simulink model "IEEE13bus_1subsystem"  (R2022b)
settings: Solver=ode4  StartTime=0.0  StopTime=inf  FixedStep=Ts  MaxStep=1e-4  RelTol=1e-4
InitFcn:
  | a=1; % Loading Factor
  | Ts=50e-6;
  | % phase to sequence conversion of RXB matrices
  | c=1*exp(sqrt(-1)*(120*pi/180));
  | T=[1 1 1;1 c*c c;1 c c*c];
  | Tinv=1/3*[1 1 1;1 c c*c;1 c*c c];
  | 
  | % Simulation data for the IEEE 13 Node Test Feeder model
  | mi2km = 1.60934;%  miles to km conversion
  | ft2km = 0.0003048; % feet to km conversion
  | ms2F = 1*1e-6/(2*pi*60);% microsiemens to Farads conversion
  | 
  | 
  | %% Configuration 601
  | % Series Resitance and Reactance - ohm/mile
  | R_601 = [0.3465 0.1560 0.1580;0.1560 0.3375 0.1535;0.1580 0.1535 0.3414];
  | X_601 = [1.1079 0.5017 0.4236;0.5017 1.0478 0.3849;0.4236 0.3849 1.0348];
  | % charging susceptance - microsiemens/mile
  | B_601 = [6.2998 -1.9958 -1.2595;-1.9958 5.9597 -0.7417;-1.2595 -0.7417 5.6386];
  | 
  | R_601 = R_601/mi2km;
  | Rseq=Tinv*R_601*T;
  | R1_601=Rseq(2,2);R0_601=Rseq(1,1);
  | 
  | L_601 = (X_601/(2*pi*60))/mi2km;
  | Lseq=Tinv*L_601*T;
  | L1_601=Lseq(2,2);L0_601=Lseq(1,1);
  | 
  | C_601 =(B_601*ms2F)/mi2km;
  | Cseq=Tinv*C_601*T;
  | C1_601=Cseq(2,2);C0_601=Cseq(1,1);
  | 
  | %% Configuration 602 - series reactance - ohm/mile
  | R_602 = [0.7526 0.1580 0.1560;0.1580 0.7475 0.1535;0.1560 0.1535 0.7436];
  | X_602 = [1.1814 0.4236 0.5017;0.4236 1.1983 0.3849;0.5017 0.3849 1.2112];
  | % charging susceptance - microsiemens/mile
  | B_602 = [5.6990 -1.0817 -1.6905;-1.0817 5.1795 -0.6588;-1.6905 -0.6588 5.4246];
  | 
  | R_602 = R_602/mi2km;
  | Rseq=Tinv*R_602*T;
  | R1_602=Rseq(2,2);R0_602=Rseq(1,1);
  | 
  | L_602 = (X_602/(2*pi*60))/mi2km;
  | Lseq=Tinv*L_602*T;
  | L1_602=Lseq(2,2);L0_602=Lseq(1,1);
  | 
  | C_602 =(B_602*ms2F)/mi2km;
  | Cseq=Tinv*C_602*T;
  | C1_602=Cseq(2,2);C0_602=Cseq(1,1);
  | %% Configuration 603 - series reactance - ohm/mile
  | R_603 = [0 0 0;0 1.3294 0.2066;0 0.2066 1.3238];
  | X_603 = [0 0 0;0 1.3471 0.4591;0 0.4591 1.3569];
  | % charging susceptance - microsiemens/mile
  | B_603 = [0 0 0;0 4.7097 -0.8999;0 -0.8999 4.6658];
  | 
  | % convert for SPS
  | R_603 = R_603/mi2km;
  | Rseq=Tinv*R_603*T;
  | R1_603=Rseq(2,2);R0_603=Rseq(1,1);
  | 
  | L_603 = (X_603/(2*pi*60))/mi2km;
  | Lseq=Tinv*L_603*T;
  | L1_603=Lseq(2,2);L0_603=Lseq(1,1);
  | 
  | C_603 =(B_603*ms2F)/mi2km;
  | Cseq=Tinv*C_603*T;
  | C1_603=Cseq(2,2);C0_603=Cseq(1,1);
  | %% Configuration 604 - series reactance - ohm/mile
  | R_604 = [1.3238 0 0.2066;0 0 0;0.2066 0 1.3294];
  | X_604 = [1.3569 0 0.4591;0 0 0;0.4591 0 1.3471];
  | % charging susceptance - microsiemens/mile
  | B_604 = [4.6658 0 -0.8999;0 0 0;-0.8999 0 4.7097];
  | R_604 = R_604/mi2km;
  | Rseq=Tinv*R_604*T;
  | R1_604=Rseq(2,2);R0_604=Rseq(1,1);
  | 
  | L_604 = (X_604/(2*pi*60))/mi2km;
  | Lseq=Tinv*L_604*T;
  | L1_604=Lseq(2,2);L0_604=Lseq(1,1);
  | 
  | C_604 =(B_604*ms2F)/mi2km;
  | Cseq=Tinv*C_604*T;
  | C1_604=Cseq(2,2);C0_604=Cseq(1,1);
  | %% Configuration 605 - series reactance - ohm/mile
  | R_605 = [0 0 0;0 0 0;0 0 1.3292];
  | X_605 = [0 0 0;0 0 0;0 0 1.3475];
  | % charging susceptance - microsiemens/mile
  | B_605 = [0 0 0;0 0 0;0 0 4.5193];
  | R_605 = R_605/mi2km;
  | Rseq=Tinv*R_605*T;
  | R1_605=Rseq(2,2);R0_605=Rseq(1,1);
  | 
  | L_605 = (X_605/(2*pi*60))/mi2km;
  | Lseq=Tinv*L_605*T;
  | L1_605=Lseq(2,2);L0_605=Lseq(1,1);
  | 
  | C_605 =(B_605*ms2F)/mi2km;
  | Cseq=Tinv*C_605*T;
  | C1_605=Cseq(2,2);C0_605=Cseq(1,1);
  | %% Configuration 606 - series reactance - ohm/mile
  | R_606 = [0.7982 0.3192 0.2849;0.3192 0.7891 0.3192;0.2849 0.3192 0.7982];
  | X_606 = [0.4463 0.0328 0.0143;0.0328 0.4041 0.0328;0.0143 0.0328 0.4463];
  | % charging susceptance - microsiemens/mile
  | B_606 = [96.8897 -1e-6 -1e-6;-1e-6 96.8897 -1e-6;-1e-6 -1e-6 96.8897];
  | R_606 = R_606/mi2km;
  | Rseq=Tinv*R_606*T;
  | R1_606=Rseq(2,2);R0_606=Rseq(1,1);
  | 
  | L_606 = (X_606/(2*pi*60))/mi2km;
  | Lseq=Tinv*L_606*T;
  | L1_606=Lseq(2,2);L0_606=Lseq(1,1);
  | 
  | C_606 =(B_606*ms2F)/mi2km;
  | Cseq=Tinv*C_606*T;
  | C1_606=Cseq(2,2);C0_606=Cseq(1,1);
  | %% Configuration 607 - series reactance - ohm/mile
  | R_607 = [1.3425 0 0;0 0 0;0 0 0];
  | X_607 = [0.5124 0 0;0 0 0;0 0 0];
  | % charging susceptance - microsiemens/mile
  | B_607 = [88.9912 0 0;0 0 0;0 0 0];
  | R_607 = R_607/mi2km;
  | Rseq=Tinv*R_607*T;
  | R1_607=Rseq(2,2);R0_607=Rseq(1,1);
  | 
  | L_607 = (X_607/(2*pi*60))/mi2km;
  | Lseq=Tinv*L_607*T;
  | L1_607=Lseq(2,2);L0_607=Lseq(1,1);
  | 
  | C_607 =(B_607*ms2F)/mi2km;
  | Cseq=Tinv*C_607*T;
  | C1_607=Cseq(2,2);C0_607=Cseq(1,1);
undefined symbols (not defined in the file): find_system, I, Left, MOV_segment9, powergui, Right, type, V, X
libraries: spsSeriesRLCBranchLib x57, spsGroundLib x42, spsVoltageMeasurementLib x18, spsThreePhaseVIMeasurementLib x16, spsDCVoltageSourceLib x12, spsThreePhaseSeriesRLCLoadLib x7, ssn_lib x6, spsACCurrentSourceLib x6, spsOnDelayLib x6, spsThreePhasePISectionLineLib x5, spsSeriesRLCLoadLib x5, spsRMSLib x4
(part 1 of 4)
settings Model: ARTEMISmethode_block_infos=$$__separator__$$IEEE13bus_1subsystem/ARTEMIS Guide$$__separator__$$  Creator=Arun  LastModifiedBy=AS7434
settings SolverCC: ShapePreserveControl=EnableAll  AlgebraicLoopSolver=TrustRegion  SolverResetMethod=Robust
settings DataIOCC: ReturnWorkspaceOutputs=off
settings DebuggingCC: SFMachineParentedDataDiag=warning  ArithmeticOperatorsInVariantConditions=warning
settings ModelReferenceCC: EnableRefExpFcnMdlSchedulingChecks=on
settings SFSimCC: SimUseLocalCustomCode=off  CustomCodeUndefinedFunction=UseInterfaceOnly
settings RTWCC: RTWUseLocalCustomCode=off
settings CodeAppCC: StateflowObjectComments=on
settings SimscapeCC: SimscapeNormalizeSystem=off

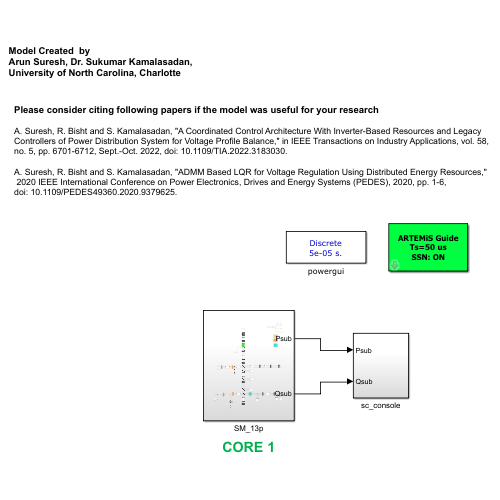
[thumbnail: Simulink's stored preview of the top-level diagram]
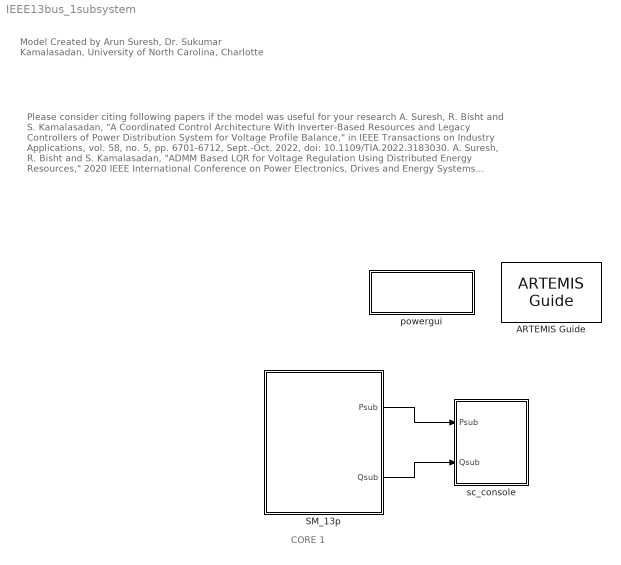
== system IEEE13bus_1subsystem ==
  note: CORE 1
  note: Please consider citing following papers if the model was useful for your research
      |
      | A. Suresh, R. Bisht and S. Kamalasadan, "A Coordinated Control Architecture With Inverter-Based Resources and Legacy
      | Controllers of Power Distribution System for Voltage Profile Balance," in IEEE Transactions on Industry Applications, vol. 58,
      | no. 5, pp. 6701-6712, Sept.-Oct. 2022, doi: 10.1109/TIA.2022.3183030.
      |
      | A. Suresh, R. Bisht and S. Kamalasadan, "ADMM Based LQR for Voltage Regulation Using Distributed Energy Resources,"
      | 2020 IEEE International Conference on Power Electronics, Drives and Energy Systems (PEDES), 2020, pp. 1-6,
      | doi: 10.1109/PEDES49360.2020.9379625.
  note: Model Created by
      | Arun Suresh, Dr. Sukumar Kamalasadan,
      | University of North Carolina, Charlotte
  ARTEMIS Guide : artemis/ARTEMIS/ARTEMIS Guide  Tag=FTSSmethode_opal_4hx0r99  Description=5.0_z1  lock=on  Ts=Ts  ssn=on  opt=art5  dyna=off  nb_perm=4  RT_fullcomp=off  ssn_itvc=off  ssn_ivic=off  ssn_ext=off  ssn_solver=Art5  iter_type=iSWITCH and iMOV only (default)  ssn_ImpulseLoopBlockedStateUpdate=5  ssn_mov_iter_number=5  ssn_switch_iter_number=5  ssn_lu_or_ldlt=LU (more robust)  ssn_nib_type_verify=on  ssn_use_lu=on  ssn_use_ldlt=off  ssn_impulse=on  ssn_quasimpulse=off  ssn_impulse_loop=5  paraExtinctionThy=off  Thy_Impulse=on  dtc=Off  dtc_opt=normal  ao=on  simtype=off  ct_mac=off  lin_mov=off  lsp=[0.001 2]  spike_skip=Disabled  dtc_extra=1  dtc_sws=normal  dtc_pied=0.5  SPSRulesBlock=SPSRules  tre=on  ctmm=off  LF=off  dpl_type=ARTEMiS DPL  rlc_type=off  custom_type=off  para=on  ssn_full_iteration=off  ssn_init_cond=block only
  SM_13p : Subsystem
  powergui : Subsystem  Priority=1  DialogController=POWERSYS.PowerSysDialog  InitFcn=powergui( 'InitFcn_Callback' , gcb , 0 , [ ] );  mask(PSB option menu block){SimulationMode=Discrete, SampleTime=Ts, frequency=60, Iterations=50, frequencyindice=0, Pbase=100e6, ErrMax=1e-4, UnitsV=kV, UnitsW=MW, buscounter=0, FunctionMessages=off, echomessages=on, EnableUseOfTLC=off, CurrentSourceSwitches=off, DisableSnubberDevices=off, DisableRonSwitches=off, DisableVfSwitches=off, DisplayEquations=off, AutomaticDiscreteSolvers=off, SolverType=Tustin, Interpol=off, ExternalGateDelay=off, methode=off, Ts=0, x0status=blocks, SPID=off, SwTol=0, HookPort=off, NonlinearTolerance=1e-4, nMaxIteration=100, ContinueOnMaxIteration=off, RestoreLinks=warning, ResistiveCurrentMeasurement=off, Frange=[0:2:500], Ylog=off, Xlog=on, ShowGrid=off, save=off, variable=ZData, structure=0, ZoomFFT=off, StartTime=0.0, cycles=1, DisplayStyle=1, fundamental=60, FreqAxis=off, MaxFrequency=1000, frequencyindicesteady=1, RmsSteady=1, display=off}
      mask prompts: SimulationMode "Simulation type:"; SampleTime "Sample time (s):"; frequency "Frequency (Hz):"; Iterations "Max iterations"; frequencyindice "Frequency (Hz)"; Pbase "Base power (VA)"; ErrMax "PQ tolerance (pu)"; UnitsV "Voltage units"; UnitsW "Power units"; buscounter "Load flow bus counter"; FunctionMessages "Disable Specialized Power Systems warnings"; echomessages "Display Specialized Power Systems compilation messages"; EnableUseOfTLC "Use TLC file when in Accelerator Simulation Mode and for code generation"; CurrentSourceSwitches "Disable ideal switching"; DisableSnubberDevices "Disable snubbers in switching devices"; DisableRonSwitches "Disable Ron resistances in switching devices"; DisableVfSwitches "Disable forward voltages in switching devices"; DisplayEquations "Display circuit differential equations"; AutomaticDiscreteSolvers "Automatically handle Discrete solver and Advanced tab solver settings of blocks"; SolverType "Discrete solver"; Interpol "Interpolate switching events"; ExternalGateDelay "Use time-stamped gate signals"; methode "Store switching topologies"; Ts "Buffer size (MBytes):"; x0status "Start simulation with initial electrical states from:"; SPID "Use ideal switching devices"; SwTol "Switch tolerance"; HookPort "Allow multiple powergui blocks"; NonlinearTolerance "Solver tolerance"; nMaxIteration "Maximum number of iterations"; ContinueOnMaxIteration "Continue Simulation if maximum number of iterations is reached"; RestoreLinks "Restore disabled links of Simscape Power Systems ST blocks:"; ResistiveCurrentMeasurement "Use non ideal current measurement blocks (1e-4Ohm internal resistance)"; Frange "Frequency Range"; Ylog "Log impedance"; Xlog "log Frequency"; ShowGrid "grid"; save "Save Data To Workspace"; variable "Variable Name"; structure "Structure Name (PSBFFTSCOPE)"; ZoomFFT "ZoomFFT (PSBFFTSCOPE)"; StartTime "Start Time (PSBFFTSCOPE)"; cycles "Cycles (PSBFFTSCOPE)"; DisplayStyle "Display style (PSBFFTSCOPE)"; fundamental "Fundamental (PSBFFTSCOPE)"; FreqAxis "Frequency Axis (PSBFFTSCOPE)"; MaxFrequency "Max Frequency (PSBFFTSCOPE)"; frequencyindicesteady "Frequency indice (STEADYSTATE)"; RmsSteady "RMS display (STEADYSTATE)"; display "Display Results"
      mask help: Set simulation type, simulation parameters, and preferences.
      mask init:
      | dispMessage = powergui('MaskInitialization',gcb,SimulationMode,SampleTime);
      settings: LibrarySourceBlock=sps_lib/powergui  PreSaveFcn=powergui( 'PreSaveFcn_Callback' , gcb , [ ] , [ ] );  OpenFcn=sps_rtmsupport('OpenFcn',gcbh)
      mask Help: helpview(psbhelp)
      mask TypeOptions SimulationMode: Continuous | Discrete | Phasor | Discrete phasor
      mask Callback SimulationMode: powergui('SimulationType',[],[],gcb);
      mask TypeOptions UnitsV: V | kV
      mask TypeOptions UnitsW: W | kW | MW
      mask Callback CurrentSourceSwitches: powergui('SimulationType',[],[],gcb);
      mask Callback AutomaticDiscreteSolvers: powergui('SimulationType',[],[],gcb);
      mask TypeOptions SolverType: Tustin/Backward Euler (TBE) | Tustin | Backward Euler
      mask Callback SolverType: powergui('SimulationType',[],[],gcb);
      mask Callback Interpol: powergui('SimulationType',[],[],gcb);
      mask Callback ExternalGateDelay: powergui('SimulationType',[],[],gcb);
      mask Callback methode: powergui('SimulationType',[],[],gcb);
      mask TypeOptions x0status: blocks | steady | zero
      mask TypeOptions RestoreLinks: yes | warning | no
      mask Callback display: sps_rtmsupport('parametereditingmodes',gcbh) % Will be executed last in parameter callbacks to ensure mask enable consistency
      mask DialogControl SolverTab Prompt: Solver
      mask DialogControl AutoSolverNote Prompt: The Simulation type parameter is governed by Simulink. To access the Powergui solver settings, unselect auto (Automatic solver selection) solver in the Simulink solver options.
      mask DialogControl Container15 Prompt: Tools
      mask DialogControl StateAnalyzer Prompt: Measurements and States Analyzer
      mask DialogControl StateAnalyzer Callback: powerStates(bdroot(gcb))
      mask DialogControl RLCLineParameters Prompt: Power Line Parameters
      mask DialogControl RLCLineParameters Callback:
      | close_system(gcb)
      | powerLineParameters
      mask DialogControl Control15 Prompt: Power Cable Parameters
      mask DialogControl Control15 Callback:
      | close_system(gcb)
      | powerCableParameters
      mask DialogControl DecouplingLines Prompt: Specify Decoupling Lines
      mask DialogControl DecouplingLines Tooltip: Click to replace selected Distributed Parameters Line blocks with Decoupling Line blocks
      mask DialogControl DecouplingLines Callback:
      | close_system(gcb);
      | DecouplingLineReplace(gcs)
      mask DialogControl LoadFlow Prompt: Load Flow Analyzer
      mask DialogControl LoadFlow Callback:
      | close_system(gcb)
      | powerLoadFlow
      mask DialogControl Container11 Prompt: Load Flow Parameters
      mask DialogControl MachineInitialization Prompt: Machine Initialization
      mask DialogControl MachineInitialization Callback:
      | close_system(gcb)
      | powericon('machineInitTool',bdroot(gcb),gcb)
      mask DialogControl ImpedanceMeasurement Prompt: Impedance Measurement
      mask DialogControl ImpedanceMeasurement Callback:
      | close_system(gcb);
      | powerImpedance(bdroot(gcs));
      mask DialogControl FFTAnalysis Prompt: FFT Analysis
      mask DialogControl FFTAnalysis Callback:
      | close_system(gcb)
      | power_fftscope(bdroot(gcb),gcb)
      mask DialogControl LinearSystemAnalyzer Prompt: Use Linear System Analyzer
      mask DialogControl LinearSystemAnalyzer Callback:
      | close_system(gcb)
      | power_ltiview(bdroot(gcb))
      mask DialogControl HysteresisDesign Prompt: Hysteresis Design
      mask DialogControl HysteresisDesign Callback:
      | close_system(gcb)
      | powerHysteresis('hysteresis.mat')
      mask DialogControl Control14 Prompt: Customize SPS blocks
      mask DialogControl Control14 Callback:
      | close_system(gcb);
      | power_customize;
      mask DialogControl GenerateReprot Prompt: Generate Report
      mask DialogControl GenerateReprot Callback:
      | close_system(gcb)
      | power_report(bdroot(gcb))
      mask DialogControl ParameterTabVar012 Prompt: Preferences
      mask DialogControl Solver Prompt: Solver
      mask DialogControl SolverDetails Prompt: Solver details for nonlinear elements
      mask Display: color('blue'),disp(dispMessage)
  sc_console : Subsystem
  wires:
  SM_13p/1(Psub) -> sc_console/1(Psub)
  SM_13p/2(Qsub) -> sc_console/2(Qsub)

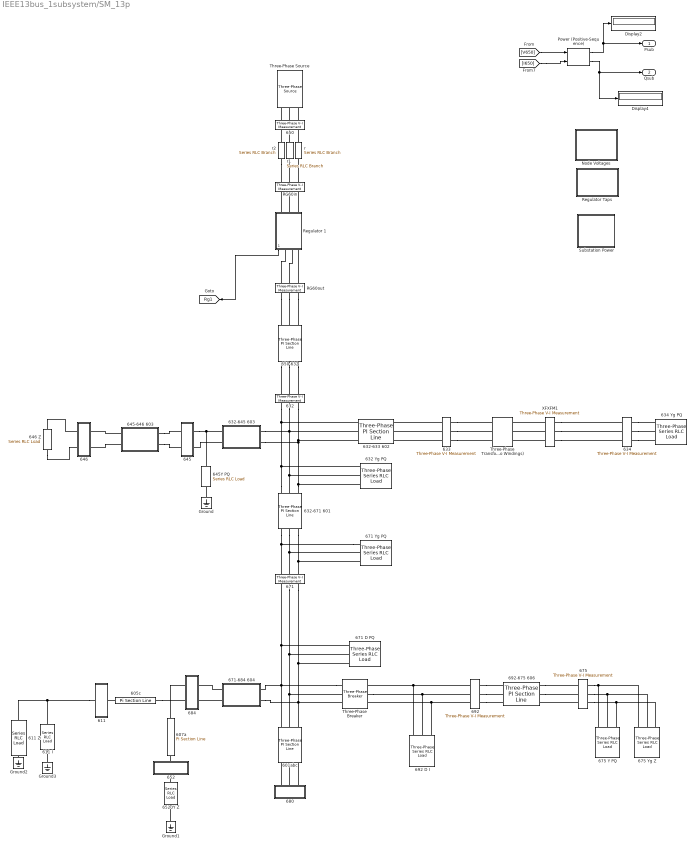
== system IEEE13bus_1subsystem/SM_13p ==
  601abc : spsThreePhasePISectionLineLib/Three-Phase PI Section Line  LConnTagsString=a|b|c  RConnTagsString=A|B|C  Length=1000*ft2km  Frequency=60  Resistances=[R1_601 R0_601]  Inductances=[L1_601 L0_601]  Capacitances=[C1_601 C0_601]
  605c : spsPiSectionLineLib/Pi Section Line  LConnTagsString=__new0  RConnTagsString=__new0  Phases=1  PiSections=1  Length=300*ft2km  Frequency=60  Resistance=R1_605  Inductance=L1_605  Capacitance=C1_605  SpecifyConductance=off  Conductance=0  Measurements=None  Measurements2=None
      settings: LibrarySourceBlock=sps_lib/Power Grid Elements/Pi Section Line
  607a : spsPiSectionLineLib/Pi Section Line  LConnTagsString=__new0  RConnTagsString=__new0  Phases=1  PiSections=1  Length=800*ft2km  Frequency=60  Resistance=R1_607  Inductance=L1_607  Capacitance=C1_607  SpecifyConductance=off  Conductance=0  Measurements=None  Measurements2=None
      settings: LibrarySourceBlock=sps_lib/Power Grid Elements/Pi Section Line
  611 : Subsystem
  611 I : spsSeriesRLCLoadLib/Series RLC Load  LConnTagsString=a  RConnTagsString=__new0  NominalVoltage=1*2401.78  NominalFrequency=60  ActivePower=170e3*a  InductivePower=80e3*a  CapacitivePower=0  Setx0=off  InitialVoltage=0  SetiL0=off  InitialCurrent=0  Measurements=None  LoadType=constant I
  611 Z : spsSeriesRLCLoadLib/Series RLC Load  LConnTagsString=a  RConnTagsString=__new0  NominalVoltage=2401.78  NominalFrequency=60  ActivePower=0  InductivePower=0  CapacitivePower=100e3*a  Setx0=off  InitialVoltage=0  SetiL0=off  InitialCurrent=0  Measurements=None  LoadType=constant Z
  632 : spsThreePhaseVIMeasurementLib/Three-Phase V-I Measurement  VoltageMeasurement=phase-to-ground  SetLabelV=on  LabelV=V632  Vpu=off  VpuLL=off  CurrentMeasurement=yes  SetLabelI=on  LabelI=I632  Ipu=off  Pbase=100e6  Vbase=24900  OutputType=Complex  PhasorSimulation=off  PSBequivalent=0
  632 Yg PQ : spsThreePhaseSeriesRLCLoadLib/Three-Phase Series RLC Load  LConnTagsString=A|B|C  Configuration=Y (grounded)  NominalVoltage=[ 1.021 1.042 1.0174]*2401.78  Vabc=[ 1 1 1]*2401.78  Vabcp=[1e3 1e3 1e3]  NominalFrequency=60  UnbalancedPower=on  ActivePower="[17 66  117]*1e3/2"  InductivePower="[10 38  68]*1e3/2"  CapacitivePower=100  Pabc="[17 66  117]*1e3/2*a"  QLabc="[10 38  68]*1e3/2*a"  QCabc=[0 0 0]  Pabcp=[10e3 9e3 11e3]  QLabcp=[100 90 110]  QCabcp=[100 90 110]  Measurements=None  LoadType=constant PQ
  632-633 602 : spsThreePhasePISectionLineLib/Three-Phase PI Section Line  LConnTagsString=a|b|c  RConnTagsString=A|B|C  Length=500*ft2km  Frequency=60  Resistances=[R1_602 R0_602]  Inductances=[L1_602 L0_602]  Capacitances=[C1_602 C0_602]
  632-645 603 : Subsystem  mask(Two-Phase PI Section Block){Rl=R_603, Ll=L_603, Cl=C_603, L=500*ft2km}
      mask prompts: Rl "Resistance per unit Length(Ohm/Km)[3x3 matrix]"; Ll "Inductance per unit Length(H/Km)[3x3 matrix]"; Cl "Capacitance per unit Length(F/Km)[3x3 matrix"; L "Length (Km)"
      mask help: This block models a two-phase transmission line with a single PI section.
      mask init:
      | W = sign(sum(abs(Rl)));
      | s = find(W==1);%Identify non zero rows and columns
      | 
      | Rt =Rl(s,s);
      | Rl= Rt;
      | Lt =Ll(s,s);
      | Ll= Lt;
      | Ct =Cl(s,s);
      | Cl= Ct;
      mask Display:
      | color('green')
      | plot(0,0,100,100,[20,20,80,80,90,80,80,20,20,10],[50,40,40,50,50,50,61,61,50,50],[56,39],[55,55],[44,44],[44,55],[53,50,50],[44,48,55])
      | color('black')
      | port_label('RConn', 1, 'b')
      | port_label('RConn', 2, 'c')
      | port_label('LConn', 1, 'B')
      | port_label('LConn', 2, 'C')
  632-671 601 : spsThreePhasePISectionLineLib/Three-Phase PI Section Line  LConnTagsString=a|b|c  RConnTagsString=A|B|C  Length=2000*ft2km  Frequency=60  Resistances=[R1_601 R0_601]  Inductances=[L1_601 L0_601]  Capacitances=[C1_601 C0_601]
  633 : spsThreePhaseVIMeasurementLib/Three-Phase V-I Measurement  VoltageMeasurement=phase-to-ground  SetLabelV=on  LabelV=V633  Vpu=off  VpuLL=off  CurrentMeasurement=no  SetLabelI=on  LabelI=I634  Ipu=off  Pbase=100e6  Vbase=24900  OutputType=Complex  PhasorSimulation=off  PSBequivalent=0
  634 : spsThreePhaseVIMeasurementLib/Three-Phase V-I Measurement  VoltageMeasurement=phase-to-ground  SetLabelV=on  LabelV=V634  Vpu=off  VpuLL=off  CurrentMeasurement=yes  SetLabelI=on  LabelI=I634  Ipu=off  Pbase=100e6  Vbase=24900  OutputType=Complex  PhasorSimulation=off  PSBequivalent=0
  634 Yg PQ : spsThreePhaseSeriesRLCLoadLib/Three-Phase Series RLC Load  LConnTagsString=A|B|C  Configuration=Y (grounded)  NominalVoltage=[ 1.021 1.042 1.0174]*2401.78  Vabc=[1 1 1]*277.128  Vabcp=[1e3 1e3 1e3]  NominalFrequency=60  UnbalancedPower=on  ActivePower="[17 66  117]*1e3/2"  InductivePower="[10 38  68]*1e3/2"  CapacitivePower=100  Pabc=[160 120 120]*1e3*a  QLabc=[110 90 90]*1e3*a  QCabc=[0 0 0]  Pabcp=[10e3 9e3 11e3]  QLabcp=[100 90 110]  QCabcp=[100 90 110]  Measurements=None  LoadType=constant PQ
  645 : Subsystem
  645-646 603 : Subsystem  mask(Two-Phase PI Section Block){Rl=R_603, Ll=L_603, Cl=C_603, L=300*ft2km}
      mask prompts: Rl "Resistance per unit Length(Ohm/Km)[3x3 matrix]"; Ll "Inductance per unit Length(H/Km)[3x3 matrix]"; Cl "Capacitance per unit Length(F/Km)[3x3 matrix"; L "Length (Km)"
      mask help: This block models a two-phase transmission line with a single PI section.
      mask init:
      | W = sign(sum(abs(Rl)));
      | s = find(W==1);%Identify non zero rows and columns
      | 
      | Rt =Rl(s,s);
      | Rl= Rt;
      | Lt =Ll(s,s);
      | Ll= Lt;
      | Ct =Cl(s,s);
      | Cl= Ct;
      mask Display:
      | color('green')
      | plot(0,0,100,100,[20,20,80,80,90,80,80,20,20,10],[50,40,40,50,50,50,61,61,50,50],[56,39],[55,55],[44,44],[44,55],[53,50,50],[44,48,55])
      | color('black')
      | port_label('RConn', 1, 'b')
      | port_label('RConn', 2, 'c')
      | port_label('LConn', 1, 'B')
      | port_label('LConn', 2, 'C')
  645Y PQ : spsSeriesRLCLoadLib/Series RLC Load  LConnTagsString=a  RConnTagsString=__new0  NominalVoltage=1*2401.78  NominalFrequency=60  ActivePower=170e3*a  InductivePower=125e3*a  CapacitivePower=0  Setx0=off  InitialVoltage=0  SetiL0=off  InitialCurrent=0  Measurements=None  LoadType=constant PQ
  646 : Subsystem
  646 Z : spsSeriesRLCLoadLib/Series RLC Load  LConnTagsString=a  RConnTagsString=__new0  NominalVoltage=4160  NominalFrequency=60  ActivePower=230e3*a  InductivePower=132e3*a  CapacitivePower=0  Setx0=off  InitialVoltage=0  SetiL0=off  InitialCurrent=0  Measurements=None  LoadType=constant Z
  650 : spsThreePhaseVIMeasurementLib/Three-Phase V-I Measurement  VoltageMeasurement=phase-to-ground  SetLabelV=on  LabelV=V650  Vpu=off  VpuLL=off  CurrentMeasurement=yes  SetLabelI=on  LabelI=I650  Ipu=off  Pbase=100e6  Vbase=24900  OutputType=Complex  PhasorSimulation=off  PSBequivalent=0
  650-632 : spsThreePhasePISectionLineLib/Three-Phase PI Section Line  LConnTagsString=a|b|c  RConnTagsString=A|B|C  Length=2000*ft2km  Frequency=60  Resistances=[R1_601 R0_601]  Inductances=[L1_601 L0_601]  Capacitances=[C1_601 C0_601]
  652 : Subsystem
  6520Y Z : spsSeriesRLCLoadLib/Series RLC Load  LConnTagsString=a  RConnTagsString=__new0  NominalVoltage=1.0*2401.78  NominalFrequency=60  ActivePower=128e3*a  InductivePower=86e3*a  CapacitivePower=0  Setx0=off  InitialVoltage=0  SetiL0=off  InitialCurrent=0  Measurements=None  LoadType=constant Z
  671 : spsThreePhaseVIMeasurementLib/Three-Phase V-I Measurement  VoltageMeasurement=phase-to-ground  SetLabelV=on  LabelV=V671  Vpu=off  VpuLL=off  CurrentMeasurement=no  SetLabelI=on  LabelI=I634  Ipu=off  Pbase=100e6  Vbase=24900  OutputType=Complex  PhasorSimulation=off  PSBequivalent=0
  671 D PQ : spsThreePhaseSeriesRLCLoadLib/Three-Phase Series RLC Load  LConnTagsString=A|B|C  Configuration=Delta  NominalVoltage=[ 1.021 1.042 1.0174]*2401.78  Vabc=[ 1.73773 1.77224 1.71484]*2401.78  Vabcp=[ 1 1 1]*4160  NominalFrequency=60  UnbalancedPower=on  ActivePower="[17 66  117]*1e3/2"  InductivePower="[10 38  68]*1e3/2"  CapacitivePower=100  Pabc=[385 385 385 ]*1e3  QLabc=[220 220 220]*1e3  QCabc=[0 0 0]  Pabcp=[385 385 385 ]*1e3*a  QLabcp=[220 220 220]*1e3*a  QCabcp="[0  0  0]"  Measurements=Branch voltages and currents  LoadType=constant PQ
  671 Yg PQ : spsThreePhaseSeriesRLCLoadLib/Three-Phase Series RLC Load  LConnTagsString=A|B|C  Configuration=Y (grounded)  NominalVoltage=[ 1.021 1.042 1.0174]*2401.78  Vabc=[ 1 1 1]*2401.78  Vabcp=[1e3 1e3 1e3]  NominalFrequency=60  UnbalancedPower=on  ActivePower="[17 66  117]*1e3/2"  InductivePower="[10 38  68]*1e3/2"  CapacitivePower=100  Pabc="[17 66  117]*1e3/2*a"  QLabc="[10 38  68]*1e3/2*a"  QCabc=[0 0 0]  Pabcp=[10e3 9e3 11e3]  QLabcp=[100 90 110]  QCabcp=[100 90 110]  Measurements=None  LoadType=constant PQ
  671-684 604 : Subsystem  mask(Two-Phase PI Section Block){Rl=R_604, Ll=L_604, Cl=C_604, L=300*ft2km}
      mask prompts: Rl "Resistance per unit Length(Ohm/Km)[3x3 matrix]"; Ll "Inductance per unit Length(H/Km)[3x3 matrix]"; Cl "Capacitance per unit Length(F/Km)[3x3 matrix"; L "Length (Km)"
      mask help: This block models a two-phase transmission line with a single PI section.
      mask init:
      | W = sign(sum(abs(Rl)));
      | s = find(W==1);%Identify non zero rows and columns
      | 
      | Rt =Rl(s,s);
      | Rl= Rt;
      | Lt =Ll(s,s);
      | Ll= Lt;
      | Ct =Cl(s,s);
      | Cl= Ct;
      mask Display:
      | color('green')
      | plot(0,0,100,100,[20,20,80,80,90,80,80,20,20,10],[50,40,40,50,50,50,61,61,50,50],[56,39],[55,55],[44,44],[44,55],[53,50,50],[44,48,55])
      | color('black')
      | port_label('RConn', 1, 'a')
      | port_label('RConn', 2, 'c')
      | port_label('LConn', 1, 'A')
      | port_label('LConn', 2, 'C')
  675 : spsThreePhaseVIMeasurementLib/Three-Phase V-I Measurement  VoltageMeasurement=phase-to-ground  SetLabelV=on  LabelV=V675  Vpu=off  VpuLL=off  CurrentMeasurement=no  SetLabelI=on  LabelI=I634  Ipu=off  Pbase=100e6  Vbase=24900  OutputType=Complex  PhasorSimulation=off  PSBequivalent=0
  675 Y PQ : spsThreePhaseSeriesRLCLoadLib/Three-Phase Series RLC Load  LConnTagsString=A|B|C  Configuration=Y (grounded)  NominalVoltage=[ 1.021 1.042 1.0174]*2401.78  Vabc=[ 1 1 1]*2401.78  Vabcp=[1e3 1e3 1e3]  NominalFrequency=60  UnbalancedPower=on  ActivePower="[17 66  117]*1e3/2"  InductivePower="[10 38  68]*1e3/2"  CapacitivePower=100  Pabc="[485  68  290]*1e3*a"  QLabc="[190  60  212]*1e3*a"  QCabc=[0 0 0]  Pabcp=[10e3 9e3 11e3]  QLabcp=[100 90 110]  QCabcp=[100 90 110]  Measurements=Branch voltages and currents  LoadType=constant PQ
  675 Yg Z : spsThreePhaseSeriesRLCLoadLib/Three-Phase Series RLC Load  LConnTagsString=A|B|C  Configuration=Y (grounded)  NominalVoltage=[ 1.021 1.042 1.0174]*2401.78  Vabc=[ 1.0 1.0 1.0]*2401.78  Vabcp=[1e3 1e3 1e3]  NominalFrequency=60  UnbalancedPower=on  ActivePower="[17 66  117]*1e3/2"  InductivePower="[10 38  68]*1e3/2"  CapacitivePower=100  Pabc=[0 0 0]  QLabc=[0 0 0]  QCabc=[200 200 200]*1e3*a  Pabcp=[10e3 9e3 11e3]  QLabcp=[100 90 110]  QCabcp=[100 90 110]  Measurements=None  LoadType=constant Z
  680 : Subsystem
  684 : Subsystem
  692 : spsThreePhaseVIMeasurementLib/Three-Phase V-I Measurement  VoltageMeasurement=phase-to-ground  SetLabelV=on  LabelV=V692  Vpu=off  VpuLL=off  CurrentMeasurement=no  SetLabelI=on  LabelI=I634  Ipu=off  Pbase=100e6  Vbase=24900  OutputType=Complex  PhasorSimulation=off  PSBequivalent=0
  692 D I : spsThreePhaseSeriesRLCLoadLib/Three-Phase Series RLC Load  LConnTagsString=A|B|C  Configuration=Delta  NominalVoltage=[ 1.021 1.042 1.0174]*2401.78  Vabc=[ 1.73488 1.75203 1.72341]*2401.78  Vabcp=[ 1.0 1.0 1.0]*4160  NominalFrequency=60  UnbalancedPower=on  ActivePower="[17 66  117]*1e3/2"  InductivePower="[10 38  68]*1e3/2"  CapacitivePower=100  Pabc="[17 66  117]*1e3/2"  QLabc="[10 38  68]*1e3/2"  QCabc=[0 0 0]  Pabcp=[1e-3 1e-3 170 ]*1e3*a  QLabcp=[0 0 151]*1e3*a  QCabcp="[0  0  0]"  Measurements=Branch voltages and currents  LoadType=constant Z
  692-675 606 : spsThreePhasePISectionLineLib/Three-Phase PI Section Line  LConnTagsString=a|b|c  RConnTagsString=A|B|C  Length=500*ft2km  Frequency=60  Resistances=[R1_606 R0_606]  Inductances=[L1_606 L0_606]  Capacitances=[C1_606 C0_606]
  Display2 : Display
  Display4 : Display
  Ground{,1..3} (4 alike) : spsGroundLib/Ground  LConnTagsString=a
  Node Voltages : Subsystem
  Power (Positive-Sequence) : spsPowerPositiveSequenceLib/Power (Positive-Sequence)  Freq=60  Vinit=[0, 0]  Iinit=[0, 0]  Ts=Ts
      settings: LibrarySourceBlock=|
      | sps_lib/Sensors and Measurements/Power
      | (Positive-Sequence)
  RG60in : spsThreePhaseVIMeasurementLib/Three-Phase V-I Measurement  VoltageMeasurement=phase-to-ground  SetLabelV=on  LabelV=RG60in  Vpu=off  VpuLL=off  CurrentMeasurement=yes  SetLabelI=on  LabelI=IRG60in  Ipu=off  Pbase=100e6  Vbase=24900  OutputType=Complex  PhasorSimulation=off  PSBequivalent=0
  RG60out : spsThreePhaseVIMeasurementLib/Three-Phase V-I Measurement  VoltageMeasurement=phase-to-ground  SetLabelV=on  LabelV=RG60out  Vpu=off  VpuLL=off  CurrentMeasurement=no  SetLabelI=on  LabelI=I650  Ipu=off  Pbase=100e6  Vbase=24900  OutputType=Complex  PhasorSimulation=off  PSBequivalent=0
  Regulator 1 : Subsystem
  "Regulator Taps " : Subsystem
  Substation Power : Subsystem
  Three-Phase Transformer (Two Windings) : spsThreePhaseTransformerTwoWindingsLib/Three-Phase Transformer (Two Windings)  Winding1Connection=Yg  Winding2Connection=Yg  CoreType=Three single-phase transformers  SetSaturation=off  Hysteresis=off  DataFile='hysteresis'  SetInitialFlux=off  Measurements=None  UNITS=pu  NominalPower=[ 500e3 , 60 ]  Winding1=[4160 0.011 0.02]  Winding2=[480 0 0]  Rm=500  Lm=500  L0=0.5  Saturation=[ 0,0 ; 0.0024,1.2 ; 1.0,1.52 ]  InitialFluxes=[ 0.8 , -0.8 , 0.7 ]  BreakLoop=off  DiscreteSolver=Trapezoidal iterative  DataType=off  TransfoNumber=1
  Three-Phase Breaker : spsThreePhaseBreakerLib/Three-Phase Breaker  InitialState=closed  SwitchA=off  SwitchB=off  SwitchC=off  SwitchTimes=[0.5 ]  External=off  BreakerResistance=0.0001  SnubberResistance=inf  SnubberCapacitance=0  Measurements=None
  Three-Phase Source : spsThreePhaseSourceLib/Three-Phase Source  InternalConnection=Yg  VoltagePhases=on  Voltage=25e3  PhaseAngle=0  Voltage_phases=[ 1.0 1.0 1.0]*2401.78  PhaseAngles_phases=[0 -120 120]  Frequency=60  NonIdealSource=off  SpecifyImpedance=off  Resistance=.001  Inductance=16.58e-6  ShortCircuitLevel=100e6  BaseVoltage=4160  XRratio=7  BusType=swing  Pref=10e3  Qref=0  Prefabc=[10e3, 10e3, 10e3]  Qrefabc=[0, 0, 0]  Qmin=-inf  Qmax=inf
  XFXFM1 : spsThreePhaseVIMeasurementLib/Three-Phase V-I Measurement  VoltageMeasurement=phase-to-ground  SetLabelV=on  LabelV=XFXFM1  Vpu=off  VpuLL=off  CurrentMeasurement=no  SetLabelI=on  LabelI=I634  Ipu=off  Pbase=100e6  Vbase=24900  OutputType=Complex  PhasorSimulation=off  PSBequivalent=0
  r : spsSeriesRLCBranchLib/Series RLC Branch  LConnTagsString=__new0  RConnTagsString=__new0  BranchType=R  Resistance=1e-6  Inductance=1e-6  SetiL0=off  InitialCurrent=0  Capacitance=1e-6  Setx0=off  InitialVoltage=0  Measurements=None
  r1 : spsSeriesRLCBranchLib/Series RLC Branch  LConnTagsString=__new0  RConnTagsString=__new0  BranchType=R  Resistance=1e-6  Inductance=1e-6  SetiL0=off  InitialCurrent=0  Capacitance=1e-6  Setx0=off  InitialVoltage=0  Measurements=None
  r2 : spsSeriesRLCBranchLib/Series RLC Branch  LConnTagsString=__new0  RConnTagsString=__new0  BranchType=R  Resistance=1e-6  Inductance=1e-6  SetiL0=off  InitialCurrent=0  Capacitance=1e-6  Setx0=off  InitialVoltage=0  Measurements=None
  Psub : Outport
  Qsub : Outport  Port=2
  tag scope: Rg1=global
  wires:
  Regulator 1/1(Tap) -> [Rg1]
  [I650] -> Power (Positive-Sequence)/2
  [V650] -> Power (Positive-Sequence)/1
  Power (Positive-Sequence)/1 -> Display2/1, Psub/1
  Power (Positive-Sequence)/2 -> Qsub/1, Display4/1
  connections:
  650/LConn1 -- Three-Phase Source/RConn1
  633/RConn2 -- Three-Phase Transformer (Two Windings)/LConn2
  675/RConn3 -- 675 Y PQ/LConn3 -- 675 Yg Z/LConn3
  671-684 604/RConn2 -- 684/RConn2
  671-684 604/LConn2 -- 601abc/LConn3 -- 671/RConn3 -- 671 D PQ/LConn3 -- Three-Phase Breaker/LConn3
  645/RConn1 -- 632-645 603/RConn1 -- 645Y PQ/LConn1
  650-632/RConn1 -- 632/LConn1
  632-645 603/LConn1 -- 632 Yg PQ/LConn2 -- 632-671 601/LConn2 -- 632-633 602/LConn2 -- 632/RConn2
  632-671 601/LConn1 -- 632 Yg PQ/LConn1 -- 632/RConn1 -- 632-633 602/LConn1
  Three-Phase Breaker/LConn1 -- 671-684 604/LConn1 -- 601abc/LConn1 -- 671/RConn1 -- 671 D PQ/LConn1
  632-671 601/LConn3 -- 632 Yg PQ/LConn3 -- 632/RConn3 -- 632-633 602/LConn3 -- 632-645 603/LConn2
  601abc/LConn2 -- Three-Phase Breaker/LConn2 -- 671/RConn2 -- 671 D PQ/LConn2
  650/LConn3 -- Three-Phase Source/RConn3
  692-675 606/RConn1 -- 675/LConn1
  692-675 606/RConn2 -- 675/LConn2
  675/RConn2 -- 675 Y PQ/LConn2 -- 675 Yg Z/LConn2
  Ground/LConn1 -- 645Y PQ/RConn1
  692/RConn3 -- 692-675 606/LConn3
  675/RConn1 -- 675 Y PQ/LConn1 -- 675 Yg Z/LConn1
  650-632/RConn2 -- 632/LConn2
  611/LConn1 -- 611 Z/LConn1 -- 611 I/LConn1
  692/LConn1 -- 692 D I/LConn1 -- Three-Phase Breaker/RConn1
  XFXFM1/RConn1 -- 634/LConn1
  671 Yg PQ/LConn1 -- 671/LConn1 -- 632-671 601/RConn1
  634/RConn1 -- 634 Yg PQ/LConn1
  652/RConn1 -- 607a/RConn1
  r1/RConn1 -- RG60in/LConn2
  633/LConn2 -- 632-633 602/RConn2
  XFXFM1/RConn2 -- 634/LConn2
  671/LConn2 -- 632-671 601/RConn2 -- 671 Yg PQ/LConn2
  633/LConn3 -- 632-633 602/RConn3
  Ground3/LConn1 -- 611 I/RConn1
  692/RConn1 -- 692-675 606/LConn1
  r2/LConn1 -- 650/RConn1
  652/LConn1 -- 6520Y Z/LConn1
  675/LConn3 -- 692-675 606/RConn3
  680/RConn2 -- 601abc/RConn2
  RG60out/LConn3 -- Regulator 1/RConn3
  633/RConn3 -- Three-Phase Transformer (Two Windings)/LConn3
  633/LConn1 -- 632-633 602/RConn1
  634/RConn2 -- 634 Yg PQ/LConn2
  684/LConn1 -- 607a/LConn1
  645-646 603/LConn2 -- 645/LConn2
  646 Z/RConn1 -- 646/LConn2
  605c/LConn1 -- 684/LConn2
  632-645 603/RConn2 -- 645/RConn2
  r/RConn1 -- RG60in/LConn3
  Regulator 1/LConn3 -- RG60in/RConn3
  692/LConn2 -- 692 D I/LConn2 -- Three-Phase Breaker/RConn2
  XFXFM1/LConn2 -- Three-Phase Transformer (Two Windings)/RConn2
  692/RConn2 -- 692-675 606/LConn2
  634/RConn3 -- 634 Yg PQ/LConn3
  633/RConn1 -- Three-Phase Transformer (Two Windings)/LConn1
  r/LConn1 -- 650/RConn3
  Regulator 1/LConn1 -- RG60in/RConn1
  XFXFM1/LConn1 -- Three-Phase Transformer (Two Windings)/RConn1
  650/LConn2 -- Three-Phase Source/RConn2
  Ground2/LConn1 -- 611 Z/RConn1
  680/RConn1 -- 601abc/RConn1
  RG60out/LConn2 -- Regulator 1/RConn2
  645-646 603/RConn2 -- 646/RConn2
  XFXFM1/LConn3 -- Three-Phase Transformer (Two Windings)/RConn3
  Regulator 1/LConn2 -- RG60in/RConn2
  680/RConn3 -- 601abc/RConn3
  692/LConn3 -- 692 D I/LConn3 -- Three-Phase Breaker/RConn3
  XFXFM1/RConn3 -- 634/LConn3
  645-646 603/RConn1 -- 646/RConn1
  671/LConn3 -- 632-671 601/RConn3 -- 671 Yg PQ/LConn3
  RG60out/RConn1 -- 650-632/LConn1
  Ground1/LConn1 -- 6520Y Z/RConn1
  RG60out/LConn1 -- Regulator 1/RConn1
  r1/LConn1 -- 650/RConn2
  646/LConn1 -- 646 Z/LConn1
  RG60out/RConn3 -- 650-632/LConn3
  r2/RConn1 -- RG60in/LConn1
  671-684 604/RConn1 -- 684/RConn1
  RG60out/RConn2 -- 650-632/LConn2
  645-646 603/LConn1 -- 645/LConn1
  605c/RConn1 -- 611/RConn1
  650-632/RConn3 -- 632/LConn3

== system IEEE13bus_1subsystem/powergui ==
  note: Graphical user interface for the analysis of
      | Simscape Power Systems (Specialized Technology) circuits.
      | Place the Powergui block in the top-level of your model and double-click
      | on it to open the GUI.
  EquivalentModel1 : Subsystem
      mask init:
      | S  = GetDataForEquivalentModel('Discrete',gcbh);
      mask Display:
      | color('red')
      | disp('EQUIVALENT CIRCUIT\nDiscrete')
  EquivalentModel2 : Subsystem
      mask init:
      | S  = GetDataForEquivalentModel('Discrete',gcbh);
      mask Display:
      | color('red')
      | disp('EQUIVALENT CIRCUIT\nDiscrete')
  EquivalentModel3 : Subsystem
      mask init:
      | S  = GetDataForEquivalentModel('Discrete',gcbh);
      mask Display:
      | color('red')
      | disp('EQUIVALENT CIRCUIT\nDiscrete')
  EquivalentModel4 : Subsystem
      mask init:
      | S  = GetDataForEquivalentModel('Discrete',gcbh);
      mask Display:
      | color('red')
      | disp('EQUIVALENT CIRCUIT\nDiscrete')
  Ground : Ground
  Terminator : Terminator
  wires:
  Ground/1 -> Terminator/1

== system IEEE13bus_1subsystem/sc_console ==
  Psub : Inport
  Qsub : Inport  Port=2
  OpComm : rtlab/OpComm  nbport=2  groupe_acq=1  subsys_rate=0  st=0  Synchronization=on  Interpolation=on  Threshold=1.0  Missed_Data=off  Sim_Time=off  Samples=off  dynSigOut=off  from_console=0  warning_done=off  writeOpCommFile=off  Offset=off
  Ps : Scope
  Qs : Scope
  wires:
  Psub/1 -> OpComm/1
  OpComm/1 -> Ps/1
  Qsub/1 -> OpComm/2
  OpComm/2 -> Qs/1

== system IEEE13bus_1subsystem/SM_13p/611 ==
  1 : spsThreePhaseVIMeasurementLib/Three-Phase V-I Measurement  VoltageMeasurement=phase-to-ground  SetLabelV=on  LabelV=V611  Vpu=off  VpuLL=off  CurrentMeasurement=no  SetLabelI=on  LabelI=I634  Ipu=off  Pbase=100e6  Vbase=24900  OutputType=Complex  PhasorSimulation=off  PSBequivalent=0
  Ground{1..2,9,12} (4 alike) : spsGroundLib/Ground  LConnTagsString=a
  c : PMIOPort  Side=Left
  C : PMIOPort  Port=2  Side=Right
  connections:
  Ground12/LConn1 -- 1/LConn2
  Ground9/LConn1 -- 1/RConn2
  1/LConn3 -- C/RConn1
  1/RConn3 -- c/RConn1
  Ground1/LConn1 -- 1/RConn1
  Ground2/LConn1 -- 1/LConn1

== system IEEE13bus_1subsystem/SM_13p/632-645 603 ==
  Config300 : spsMutualInductanceLib/Mutual Inductance  LConnTagsString=a|b  RConnTagsString=A|B  TypeOfMutual=Generalized mutual inductance  NumberOfWindings=2  SelfImpedance1=[1.1 1.1e-03]  SelfImpedance2=[ 1.1 1.1e-03]  ThreeWindings=on  SelfImpedance3=[ 1.1 1.1e-03]  MutualImpedance=[1.0 1.0e-03]  InductanceMatrix=Ll* L  ResistanceMatrix=Rl* L  Measurements=None
      settings: LibrarySourceBlock=sps_lib/Passives/Mutual Inductance
  Ground{2..3,5..6} (4 alike) : spsGroundLib/Ground  LConnTagsString=a
  Series RLC Branch : spsSeriesRLCBranchLib/Series RLC Branch  LConnTagsString=__new0  RConnTagsString=__new0  BranchType=C  Resistance=1  Inductance=1e-3  SetiL0=off  InitialCurrent=0  Capacitance=Cl(1,2)/2*L  Setx0=off  InitialVoltage=0  Measurements=None
  Series RLC Branch1 : spsSeriesRLCBranchLib/Series RLC Branch  LConnTagsString=__new0  RConnTagsString=__new0  BranchType=C  Resistance=1  Inductance=1e-3  SetiL0=off  InitialCurrent=0  Capacitance=Cl(1,2)/2*L  Setx0=off  InitialVoltage=0  Measurements=None
  Series RLC Branch11 : spsSeriesRLCBranchLib/Series RLC Branch  LConnTagsString=__new0  RConnTagsString=__new0  BranchType=C  Resistance=1  Inductance=1e-3  SetiL0=off  InitialCurrent=0  Capacitance=Cl(1,1)/2*L  Setx0=off  InitialVoltage=0  Measurements=None
  Series RLC Branch2 : spsSeriesRLCBranchLib/Series RLC Branch  LConnTagsString=__new0  RConnTagsString=__new0  BranchType=C  Resistance=1  Inductance=1e-3  SetiL0=off  InitialCurrent=0  Capacitance=Cl(1,1)/2*L  Setx0=off  InitialVoltage=0  Measurements=None
  Series RLC Branch3 : spsSeriesRLCBranchLib/Series RLC Branch  LConnTagsString=__new0  RConnTagsString=__new0  BranchType=C  Resistance=1  Inductance=1e-3  SetiL0=off  InitialCurrent=0  Capacitance=Cl(2,2)/2*L  Setx0=off  InitialVoltage=0  Measurements=None
  Series RLC Branch9 : spsSeriesRLCBranchLib/Series RLC Branch  LConnTagsString=__new0  RConnTagsString=__new0  BranchType=C  Resistance=1  Inductance=1e-3  SetiL0=off  InitialCurrent=0  Capacitance=Cl(2,2)/2*L  Setx0=off  InitialVoltage=0  Measurements=None
  B In : PMIOPort  Side=Left
  C in : PMIOPort  Port=2  Side=Left
  B Out : PMIOPort  Port=3  Side=Right
  C Out : PMIOPort  Port=4  Side=Right
  connections:
  Config300/LConn1 -- Series RLC Branch/LConn1 -- B In/RConn1 -- Series RLC Branch11/LConn1
  Config300/RConn1 -- Series RLC Branch2/LConn1 -- Series RLC Branch1/LConn1 -- B Out/RConn1
  Config300/LConn2 -- Series RLC Branch9/LConn1 -- Series RLC Branch/RConn1 -- C in/RConn1
  Config300/RConn2 -- Series RLC Branch3/LConn1 -- Series RLC Branch1/RConn1 -- C Out/RConn1
  Ground3/LConn1 -- Series RLC Branch11/RConn1
  Ground6/LConn1 -- Series RLC Branch9/RConn1
  Series RLC Branch3/RConn1 -- Ground5/LConn1
  Series RLC Branch2/RConn1 -- Ground2/LConn1

== system IEEE13bus_1subsystem/SM_13p/645 ==
  1 : spsThreePhaseVIMeasurementLib/Three-Phase V-I Measurement  VoltageMeasurement=phase-to-ground  SetLabelV=on  LabelV=V645  Vpu=off  VpuLL=off  CurrentMeasurement=no  SetLabelI=on  LabelI=I634  Ipu=off  Pbase=100e6  Vbase=24900  OutputType=Complex  PhasorSimulation=off  PSBequivalent=0
  Ground12 : spsGroundLib/Ground  LConnTagsString=a
  Ground9 : spsGroundLib/Ground  LConnTagsString=a
  B : PMIOPort  Side=Right
  b : PMIOPort  Port=2  Side=Left
  c : PMIOPort  Port=3  Side=Left
  C : PMIOPort  Port=4  Side=Right
  connections:
  Ground12/LConn1 -- 1/LConn1
  1/LConn3 -- C/RConn1
  1/LConn2 -- B/RConn1
  Ground9/LConn1 -- 1/RConn1
  1/RConn2 -- b/RConn1
  1/RConn3 -- c/RConn1

== system IEEE13bus_1subsystem/SM_13p/645-646 603 ==
  Config300 : spsMutualInductanceLib/Mutual Inductance  LConnTagsString=a|b  RConnTagsString=A|B  TypeOfMutual=Generalized mutual inductance  NumberOfWindings=2  SelfImpedance1=[1.1 1.1e-03]  SelfImpedance2=[ 1.1 1.1e-03]  ThreeWindings=on  SelfImpedance3=[ 1.1 1.1e-03]  MutualImpedance=[1.0 1.0e-03]  InductanceMatrix=Ll* L  ResistanceMatrix=Rl* L  Measurements=None
      settings: LibrarySourceBlock=sps_lib/Passives/Mutual Inductance
  Ground{2..3,5..6} (4 alike) : spsGroundLib/Ground  LConnTagsString=a
  Series RLC Branch : spsSeriesRLCBranchLib/Series RLC Branch  LConnTagsString=__new0  RConnTagsString=__new0  BranchType=C  Resistance=1  Inductance=1e-3  SetiL0=off  InitialCurrent=0  Capacitance=Cl(1,2)/2*L  Setx0=off  InitialVoltage=0  Measurements=None
  Series RLC Branch1 : spsSeriesRLCBranchLib/Series RLC Branch  LConnTagsString=__new0  RConnTagsString=__new0  BranchType=C  Resistance=1  Inductance=1e-3  SetiL0=off  InitialCurrent=0  Capacitance=Cl(1,2)/2*L  Setx0=off  InitialVoltage=0  Measurements=None
  Series RLC Branch11 : spsSeriesRLCBranchLib/Series RLC Branch  LConnTagsString=__new0  RConnTagsString=__new0  BranchType=C  Resistance=1  Inductance=1e-3  SetiL0=off  InitialCurrent=0  Capacitance=Cl(1,1)/2*L  Setx0=off  InitialVoltage=0  Measurements=None
  Series RLC Branch2 : spsSeriesRLCBranchLib/Series RLC Branch  LConnTagsString=__new0  RConnTagsString=__new0  BranchType=C  Resistance=1  Inductance=1e-3  SetiL0=off  InitialCurrent=0  Capacitance=Cl(1,1)/2*L  Setx0=off  InitialVoltage=0  Measurements=None
  Series RLC Branch3 : spsSeriesRLCBranchLib/Series RLC Branch  LConnTagsString=__new0  RConnTagsString=__new0  BranchType=C  Resistance=1  Inductance=1e-3  SetiL0=off  InitialCurrent=0  Capacitance=Cl(2,2)/2*L  Setx0=off  InitialVoltage=0  Measurements=None
  Series RLC Branch9 : spsSeriesRLCBranchLib/Series RLC Branch  LConnTagsString=__new0  RConnTagsString=__new0  BranchType=C  Resistance=1  Inductance=1e-3  SetiL0=off  InitialCurrent=0  Capacitance=Cl(2,2)/2*L  Setx0=off  InitialVoltage=0  Measurements=None
  B In : PMIOPort  Side=Left
  C in : PMIOPort  Port=2  Side=Left
  B Out : PMIOPort  Port=3  Side=Right
  C Out : PMIOPort  Port=4  Side=Right
  connections:
  Series RLC Branch2/RConn1 -- Ground2/LConn1
  Series RLC Branch3/RConn1 -- Ground5/LConn1
  Ground6/LConn1 -- Series RLC Branch9/RConn1
  Ground3/LConn1 -- Series RLC Branch11/RConn1
  C Out/RConn1 -- Series RLC Branch1/RConn1 -- Series RLC Branch3/LConn1 -- Config300/RConn2
  C in/RConn1 -- Series RLC Branch/RConn1 -- Series RLC Branch9/LConn1 -- Config300/LConn2
  B Out/RConn1 -- Series RLC Branch1/LConn1 -- Series RLC Branch2/LConn1 -- Config300/RConn1
  Series RLC Branch11/LConn1 -- B In/RConn1 -- Series RLC Branch/LConn1 -- Config300/LConn1

== system IEEE13bus_1subsystem/SM_13p/646 ==
  1 : spsThreePhaseVIMeasurementLib/Three-Phase V-I Measurement  VoltageMeasurement=phase-to-ground  SetLabelV=on  LabelV=V646  Vpu=off  VpuLL=off  CurrentMeasurement=no  SetLabelI=on  LabelI=I634  Ipu=off  Pbase=100e6  Vbase=24900  OutputType=Complex  PhasorSimulation=off  PSBequivalent=0
  Ground12 : spsGroundLib/Ground  LConnTagsString=a
  Ground9 : spsGroundLib/Ground  LConnTagsString=a
  B : PMIOPort  Side=Right
  b : PMIOPort  Port=2  Side=Left
  c : PMIOPort  Port=3  Side=Left
  C : PMIOPort  Port=4  Side=Right
  connections:
  1/RConn3 -- c/RConn1
  1/RConn2 -- b/RConn1
  Ground9/LConn1 -- 1/RConn1
  1/LConn2 -- B/RConn1
  1/LConn3 -- C/RConn1
  Ground12/LConn1 -- 1/LConn1

== system IEEE13bus_1subsystem/SM_13p/652 ==
  1 : spsThreePhaseVIMeasurementLib/Three-Phase V-I Measurement  VoltageMeasurement=phase-to-ground  SetLabelV=on  LabelV=V652  Vpu=off  VpuLL=off  CurrentMeasurement=no  SetLabelI=on  LabelI=I634  Ipu=off  Pbase=100e6  Vbase=24900  OutputType=Complex  PhasorSimulation=off  PSBequivalent=0
  Ground{1..2,9,12} (4 alike) : spsGroundLib/Ground  LConnTagsString=a
  a : PMIOPort  Side=Left
  A : PMIOPort  Port=2  Side=Right
  connections:
  Ground9/LConn1 -- 1/RConn2
  Ground12/LConn1 -- 1/LConn2
  Ground2/LConn1 -- 1/LConn3
  Ground1/LConn1 -- 1/RConn3
  A/RConn1 -- 1/LConn1
  a/RConn1 -- 1/RConn1

== system IEEE13bus_1subsystem/SM_13p/671-684 604 ==
  Config300 : spsMutualInductanceLib/Mutual Inductance  LConnTagsString=a|b  RConnTagsString=A|B  TypeOfMutual=Generalized mutual inductance  NumberOfWindings=2  SelfImpedance1=[1.1 1.1e-03]  SelfImpedance2=[ 1.1 1.1e-03]  ThreeWindings=on  SelfImpedance3=[ 1.1 1.1e-03]  MutualImpedance=[1.0 1.0e-03]  InductanceMatrix=Ll* L  ResistanceMatrix=Rl* L  Measurements=None
      settings: LibrarySourceBlock=sps_lib/Passives/Mutual Inductance
  Ground{2..3,5..6} (4 alike) : spsGroundLib/Ground  LConnTagsString=a
  Series RLC Branch : spsSeriesRLCBranchLib/Series RLC Branch  LConnTagsString=__new0  RConnTagsString=__new0  BranchType=C  Resistance=1  Inductance=1e-3  SetiL0=off  InitialCurrent=0  Capacitance=Cl(1,2)/2*L  Setx0=off  InitialVoltage=0  Measurements=None
  Series RLC Branch1 : spsSeriesRLCBranchLib/Series RLC Branch  LConnTagsString=__new0  RConnTagsString=__new0  BranchType=C  Resistance=1  Inductance=1e-3  SetiL0=off  InitialCurrent=0  Capacitance=Cl(1,2)/2*L  Setx0=off  InitialVoltage=0  Measurements=None
  Series RLC Branch11 : spsSeriesRLCBranchLib/Series RLC Branch  LConnTagsString=__new0  RConnTagsString=__new0  BranchType=C  Resistance=1  Inductance=1e-3  SetiL0=off  InitialCurrent=0  Capacitance=Cl(1,1)/2*L  Setx0=off  InitialVoltage=0  Measurements=None
  Series RLC Branch2 : spsSeriesRLCBranchLib/Series RLC Branch  LConnTagsString=__new0  RConnTagsString=__new0  BranchType=C  Resistance=1  Inductance=1e-3  SetiL0=off  InitialCurrent=0  Capacitance=Cl(1,1)/2*L  Setx0=off  InitialVoltage=0  Measurements=None
  Series RLC Branch3 : spsSeriesRLCBranchLib/Series RLC Branch  LConnTagsString=__new0  RConnTagsString=__new0  BranchType=C  Resistance=1  Inductance=1e-3  SetiL0=off  InitialCurrent=0  Capacitance=Cl(2,2)/2*L  Setx0=off  InitialVoltage=0  Measurements=None
  Series RLC Branch9 : spsSeriesRLCBranchLib/Series RLC Branch  LConnTagsString=__new0  RConnTagsString=__new0  BranchType=C  Resistance=1  Inductance=1e-3  SetiL0=off  InitialCurrent=0  Capacitance=Cl(2,2)/2*L  Setx0=off  InitialVoltage=0  Measurements=None
  A In : PMIOPort  Side=Left
  C in : PMIOPort  Port=2  Side=Left
  A Out : PMIOPort  Port=3  Side=Right
  C Out : PMIOPort  Port=4  Side=Right
  connections:
  Series RLC Branch2/RConn1 -- Ground2/LConn1
  Series RLC Branch3/RConn1 -- Ground5/LConn1
  Ground6/LConn1 -- Series RLC Branch9/RConn1
  Ground3/LConn1 -- Series RLC Branch11/RConn1
  Series RLC Branch3/LConn1 -- Config300/RConn2 -- C Out/RConn1 -- Series RLC Branch1/RConn1
  C in/RConn1 -- Series RLC Branch/RConn1 -- Series RLC Branch9/LConn1 -- Config300/LConn2
  Series RLC Branch2/LConn1 -- Config300/RConn1 -- A Out/RConn1 -- Series RLC Branch1/LConn1
  Series RLC Branch11/LConn1 -- A In/RConn1 -- Series RLC Branch/LConn1 -- Config300/LConn1

== system IEEE13bus_1subsystem/SM_13p/680 ==
  1 : spsThreePhaseVIMeasurementLib/Three-Phase V-I Measurement  VoltageMeasurement=phase-to-ground  SetLabelV=on  LabelV=V680  Vpu=off  VpuLL=off  CurrentMeasurement=yes  SetLabelI=on  LabelI=I680  Ipu=off  Pbase=100e6  Vbase=24900  OutputType=Complex  PhasorSimulation=off  PSBequivalent=0
  A : PMIOPort  Side=Right
  B : PMIOPort  Port=2  Side=Right
  C : PMIOPort  Port=3  Side=Right
  connections:
  1/LConn1 -- A/RConn1
  1/LConn2 -- B/RConn1
  C/RConn1 -- 1/LConn3

== system IEEE13bus_1subsystem/SM_13p/684 ==
  1 : spsThreePhaseVIMeasurementLib/Three-Phase V-I Measurement  VoltageMeasurement=phase-to-ground  SetLabelV=on  LabelV=V684  Vpu=off  VpuLL=off  CurrentMeasurement=no  SetLabelI=on  LabelI=I634  Ipu=off  Pbase=100e6  Vbase=24900  OutputType=Complex  PhasorSimulation=off  PSBequivalent=0
  Ground12 : spsGroundLib/Ground  LConnTagsString=a
  Ground9 : spsGroundLib/Ground  LConnTagsString=a
  A : PMIOPort  Side=Right
  a : PMIOPort  Port=2  Side=Left
  c : PMIOPort  Port=3  Side=Left
  C : PMIOPort  Port=4  Side=Right
  connections:
  1/RConn3 -- c/RConn1
  1/LConn3 -- C/RConn1
  Ground9/LConn1 -- 1/RConn2
  a/RConn1 -- 1/RConn1
  Ground12/LConn1 -- 1/LConn2
  1/LConn1 -- A/RConn1

== system IEEE13bus_1subsystem/SM_13p/Node Voltages ==
  Gain1 : Gain  Gain=1/(4160/sqrt(3))
  Gain3 : Gain  Gain=4160/480
  Gain4 : Gain  Gain=4160/480
  Mux : Mux  Inputs=15
  RMS : spsRMSLib/RMS  TrueRMS=on  Freq=60  RMSInit=120  Ts=0
  To Workspace : ToWorkspace  VariableName=V13  SampleTime=.1
  wires:
  RMS/1 -> Gain1/1
  Gain1/1 -> To Workspace/1
  Mux/1 -> RMS/1
  [V634] -> Gain3/1
  [V684] -> Mux/11
  [V675] -> Mux/15
  [V646] -> Mux/8
  [V633] -> Mux/4
  Gain3/1 -> Mux/6
  [XFXFM1] -> Gain4/1
  [V611] -> Mux/12
  [V632] -> Mux/3
  [V671] -> Mux/9
  [V680] -> Mux/10
  [V650] -> Mux/1
  [V652] -> Mux/13
  [RG60out] -> Mux/2
  [V692] -> Mux/14
  [V645] -> Mux/7
  Gain4/1 -> Mux/5
